simulink model "controller_sim"  (R2022a)
settings: Solver=ode1  StartTime=0.0  StopTime=10.0  FixedStep=0.010  RelTol=1e-5  AbsTol=1e-5
undefined symbols (not defined in the file or in its folder): c_d, c_dn, c_downbound, c_i, c_n, c_p, c_upbound, T0, T1, Td, Tg, Ti, Ts, Tsp, Tsp_delay, Tt
libraries: slpidlib x1
(part 1 of 3)
settings Model: Creator=baikp  LastModifiedBy=fxq001
settings SolverCC: AlgebraicLoopSolver=TrustRegion
settings DebuggingCC: UnconnectedInputMsg=warning  UnconnectedOutputMsg=warning  UnconnectedLineMsg=warning  SFMachineParentedDataDiag=warning
settings RTWCC: DLArmComputeVersion=19.05

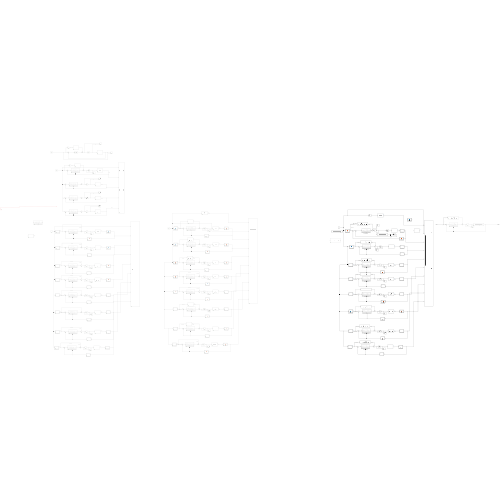
[thumbnail: Simulink's stored preview of the top-level diagram]
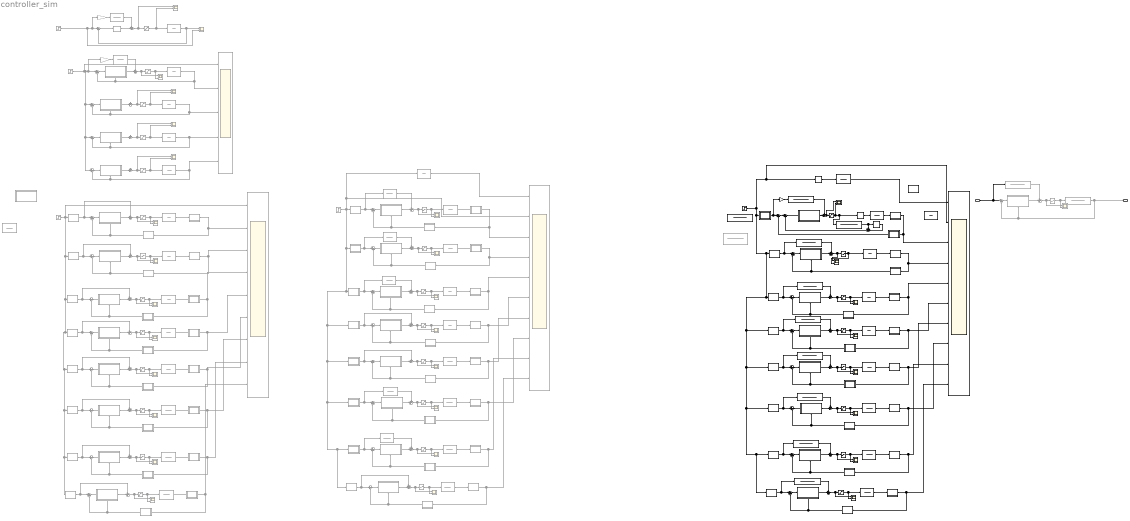
== system controller_sim ==
  In1 : Inport
  013throttle2wrpm1 : MATLAB Function  Commented=on  TreatAsAtomicUnit=on
  013throttle2wrpm2 : MATLAB Function  Commented=on  TreatAsAtomicUnit=on
  013throttle2wrpm3 : MATLAB Function  TreatAsAtomicUnit=on
  013wrpm2throttle2 : MATLAB Function  Commented=on  TreatAsAtomicUnit=on
  013wrpm2throttle3 : MATLAB Function  Commented=on  TreatAsAtomicUnit=on
  015throttle2wrpm1 : MATLAB Function  Commented=on  TreatAsAtomicUnit=on
  015throttle2wrpm2 : MATLAB Function  Commented=on  TreatAsAtomicUnit=on
  015throttle2wrpm3 : MATLAB Function  TreatAsAtomicUnit=on
  015wrpm2throttle1 : MATLAB Function  Commented=on  TreatAsAtomicUnit=on
  015wrpm2throttle4 : MATLAB Function  Commented=on  TreatAsAtomicUnit=on
  426throttle2wrpm1 : MATLAB Function  Commented=on  TreatAsAtomicUnit=on
  426throttle2wrpm2 : MATLAB Function  Commented=on  TreatAsAtomicUnit=on
  426throttle2wrpm3 : MATLAB Function  TreatAsAtomicUnit=on
  426wrpm2throttle2 : MATLAB Function  Commented=on  TreatAsAtomicUnit=on
  426wrpm2throttle3 : MATLAB Function  Commented=on  TreatAsAtomicUnit=on
  427throttle2wrpm1 : MATLAB Function  Commented=on  TreatAsAtomicUnit=on
  427throttle2wrpm2 : MATLAB Function  Commented=on  TreatAsAtomicUnit=on
  427throttle2wrpm3 : MATLAB Function  TreatAsAtomicUnit=on
  427wrpm2throttle1 : MATLAB Function  Commented=on  TreatAsAtomicUnit=on
  427wrpm2throttle10 : MATLAB Function  Commented=on  TreatAsAtomicUnit=on
  427wrpm2throttle11 : MATLAB Function  Commented=on  TreatAsAtomicUnit=on
  427wrpm2throttle12 : MATLAB Function  Commented=on  TreatAsAtomicUnit=on
  427wrpm2throttle13 : MATLAB Function  Commented=on  TreatAsAtomicUnit=on
  427wrpm2throttle14 : MATLAB Function  Commented=on  TreatAsAtomicUnit=on
  427wrpm2throttle15 : MATLAB Function  Commented=on  TreatAsAtomicUnit=on
  427wrpm2throttle16 : MATLAB Function  Commented=on  TreatAsAtomicUnit=on
  427wrpm2throttle17 : MATLAB Function  Commented=on  TreatAsAtomicUnit=on
  427wrpm2throttle18 : MATLAB Function  Commented=on  TreatAsAtomicUnit=on
  427wrpm2throttle19 : MATLAB Function  TreatAsAtomicUnit=on
  427wrpm2throttle2 : MATLAB Function  Commented=on  TreatAsAtomicUnit=on
  427wrpm2throttle20 : MATLAB Function  TreatAsAtomicUnit=on
  427wrpm2throttle21 : MATLAB Function  TreatAsAtomicUnit=on
  427wrpm2throttle22 : MATLAB Function  TreatAsAtomicUnit=on
  427wrpm2throttle23 : MATLAB Function  TreatAsAtomicUnit=on
  427wrpm2throttle24 : MATLAB Function  TreatAsAtomicUnit=on
  427wrpm2throttle25 : MATLAB Function  TreatAsAtomicUnit=on
  427wrpm2throttle26 : MATLAB Function  TreatAsAtomicUnit=on
  427wrpm2throttle27 : MATLAB Function  TreatAsAtomicUnit=on
  427wrpm2throttle28 : MATLAB Function  TreatAsAtomicUnit=on
  427wrpm2throttle29 : MATLAB Function  TreatAsAtomicUnit=on
  427wrpm2throttle3 : MATLAB Function  Commented=on  TreatAsAtomicUnit=on
  427wrpm2throttle30 : MATLAB Function  TreatAsAtomicUnit=on
  427wrpm2throttle31 : MATLAB Function  TreatAsAtomicUnit=on
  427wrpm2throttle32 : MATLAB Function  TreatAsAtomicUnit=on
  427wrpm2throttle33 : MATLAB Function  TreatAsAtomicUnit=on
  427wrpm2throttle34 : MATLAB Function  TreatAsAtomicUnit=on
  427wrpm2throttle4 : MATLAB Function  Commented=on  TreatAsAtomicUnit=on
  427wrpm2throttle5 : MATLAB Function  Commented=on  TreatAsAtomicUnit=on
  427wrpm2throttle6 : MATLAB Function  Commented=on  TreatAsAtomicUnit=on
  427wrpm2throttle7 : MATLAB Function  Commented=on  TreatAsAtomicUnit=on
  427wrpm2throttle8 : MATLAB Function  Commented=on  TreatAsAtomicUnit=on
  427wrpm2throttle9 : MATLAB Function  Commented=on  TreatAsAtomicUnit=on
  428throttle2wrpm1 : MATLAB Function  Commented=on  TreatAsAtomicUnit=on
  428throttle2wrpm2 : MATLAB Function  Commented=on  TreatAsAtomicUnit=on
  428throttle2wrpm3 : MATLAB Function  TreatAsAtomicUnit=on
  428throttle2wrpm4 : MATLAB Function  TreatAsAtomicUnit=on
  428wrpm2throttle2 : MATLAB Function  Commented=on  TreatAsAtomicUnit=on
  428wrpm2throttle3 : MATLAB Function  Commented=on  TreatAsAtomicUnit=on
  429throttle2wrpm1 : MATLAB Function  Commented=on  TreatAsAtomicUnit=on
  429throttle2wrpm2 : MATLAB Function  Commented=on  TreatAsAtomicUnit=on
  429throttle2wrpm3 : MATLAB Function  TreatAsAtomicUnit=on
  429wrpm2throttle1 : MATLAB Function  Commented=on  TreatAsAtomicUnit=on
  429wrpm2throttle4 : MATLAB Function  Commented=on  TreatAsAtomicUnit=on
  430throttle2wrpm1 : MATLAB Function  Commented=on  TreatAsAtomicUnit=on
  430throttle2wrpm2 : MATLAB Function  Commented=on  TreatAsAtomicUnit=on
  430throttle2wrpm3 : MATLAB Function  TreatAsAtomicUnit=on
  430wrpm2throttle2 : MATLAB Function  Commented=on  TreatAsAtomicUnit=on
  430wrpm2throttle3 : MATLAB Function  Commented=on  TreatAsAtomicUnit=on
  431throttle2wrpm : MATLAB Function  Commented=on  TreatAsAtomicUnit=on
  431throttle2wrpm1 : MATLAB Function  Commented=on  TreatAsAtomicUnit=on
  431throttle2wrpm2 : MATLAB Function  TreatAsAtomicUnit=on
  431wrpm2throttle : MATLAB Function  Commented=on  TreatAsAtomicUnit=on
  431wrpm2throttle1 : MATLAB Function  Commented=on  TreatAsAtomicUnit=on
  Discrete Transfer Fcn1 : DiscreteTransferFcn  Numerator=[Ts Ts]  Denominator=[(Ts+2*Tg) (Ts-2*Tg)]
  Discrete Transfer Fcn10 : DiscreteTransferFcn  Commented=on  Numerator=[Ts Ts]  Denominator=[(Ts+0.3) (Ts-0.3)]
  Discrete Transfer Fcn11 : DiscreteTransferFcn  Commented=on  Numerator=[Ts Ts]  Denominator=[(Ts+0.4) (Ts-0.4)]
  Discrete Transfer Fcn12 : DiscreteTransferFcn  Commented=on  Numerator=[(2*T0+Ts) (Ts-2*T0)]  Denominator=[(2*T1+Ts ) (Ts-2*T1)]
  Discrete Transfer Fcn{2..8,13} (8 alike) : DiscreteTransferFcn  Numerator=[Ts Ts]  Denominator=[(Ts+0.3) (Ts-0.3)]
  Discrete Transfer Fcn9 : DiscreteTransferFcn  Numerator=[Ts Ts]  Denominator=[(Ts+2*Tsp) (Ts-2*Tsp)]
  Gain : Gain  Commented=on  Gain=0.0012
  Gain1 : Gain  Commented=on  Gain=0.0012
  Gain2 : Gain  Gain=0.8
  PID Controller : slpidlib/PID Controller  Commented=on  Controller=PID  Form=Parallel  TimeDomain=Continuous-time  UseExternalTs=off  SampleTime=-1  IntegratorMethod=Forward Euler  FilterMethod=Forward Euler  ControllerParametersSource=internal  P=27.5*0.5  I=84.7*0.5  UseKiTs=off  D=2.2*0.5  N=100  UseFilter=on  TunerSelectOption=Transfer Function Based (PID Tuner App)  InitialConditionSource=internal  InitialConditionForIntegrator=0  InitialConditionForFilter=0  DifferentiatorICPrevScaledInput=0  ExternalReset=none  TrackingMode=off  Kt=1  LimitOutput=on  SatLimitsSource=internal  UpperSaturationLimit=200  LowerSaturationLimit=0  LinearizeAsGain=on  AntiWindupMode=back-calculation  Kb=4  POutMin=[]  POutMax=[]  IOutMin=[]  IOutMax=[]  DOutMin=[]  DOutMax=[]  NOutMin=[]  NOutMax=[]  SumOutMin=[]  SumOutMax=[]  SaturationOutMin=[]  SaturationOutMax=[]  PParamMin=[]  PParamMax=[]  IParamMin=[]  IParamMax=[]  DParamMin=[]  DParamMax=[]  NParamMin=[]  NParamMax=[]  KbParamMin=[]  KbParamMax=[]  KtParamMin=[]  KtParamMax=[]  KbOutMin=[]  KbOutMax=[]  KtOutMin=[]  KtOutMax=[]  IntegratorOutMin=[]  IntegratorOutMax=[]  FilterOutMin=[]  FilterOutMax=[]  SumI1OutMin=[]  SumI1OutMax=[]  SumI2OutMin=[]  SumI2OutMax=[]  SumI3OutMin=[]  SumI3OutMax=[]  SumI4OutMin=[]  SumI4OutMax=[]  SumDOutMin=[]  SumDOutMax=[]  DifferentiatorOutMin=[]  DifferentiatorOutMax=[]  FilterDiffOutCoefMin=[]  FilterDiffOutCoefMax=[]  ReciprocalOutMin=[]  ReciprocalOutMax=[]  SumDenOutMin=[]  SumDenOutMax=[]  SumNumOutMin=[]  SumNumOutMax=[]  DivideOutMin=[]  DivideOutMax=[]  UdiffTsProdOutMin=[]  UdiffTsProdOutMax=[]  NTsProdOutMin=[]  NTsProdOutMax=[]  UintegralTsProdOutMin=[]  UintegralTsProdOutMax=[]  UngainTsProdOutMin=[]  UngainTsProdOutMax=[]  IntegratorContinuousStateAttributes=''  IntegratorStateMustResolveToSignalObject=off  IntegratorRTWStateStorageClass=Auto  FilterContinuousStateAttributes=''  FilterStateMustResolveToSignalObject=off  FilterRTWStateStorageClass=Auto  ParallelPVariant=InternalParameters  IdealPVariant=Disabled  IVariant=InternalParameters  DVariant=InternalParameters  IntegratorVariant=Continuous  SatVariant=Enabled  AWVariant=BackCalculation  PCopyVariant=Disabled  TRVariant=Disabled  FdbkBlocksVariant=Forward  IdealPFdbkVariant=Disabled  SatFdbkVariant=Disabled  DerivativeFilterVariant=ContFilter  NVariant=InternalParameters  NCopyVariant=Disabled  FilterICVariant=InternalICsFilter  IntegratorICVariant=InternalICs  ExternalResetVariant=Disabled  TRSumVariant=Passthrough  SumFdbkVariant=Disabled  SumVariant=Sum_PID  TsampFilterVariant=InternalTs  TsampNgainVariant=Passthrough  TsampIntegralVariant=Passthrough  ExternalSaturationOutDataTypeStr=Inherit: Same as second input  aMode=0
  Saturation{,1..20,29} (22 alike) : Saturate  Commented=on  UpperLimit=1000  LowerLimit=0
  Saturation{21..28} (8 alike) : Saturate  UpperLimit=1000  LowerLimit=0
  Scope{,1,3..7,9..22,24,35} (23 alike) : Scope  Commented=on  NumInputPorts=2
  Scope2 : Scope  Commented=on  NumInputPorts=5
  Scope23 : Scope  Commented=on  NumInputPorts=10
  Scope{25..31,33} (8 alike) : Scope  NumInputPorts=2
  Scope32 : Scope  NumInputPorts=10
  Scope8 : Scope  Commented=on  NumInputPorts=9
  Step : Step  Commented=on  After=100  SampleTime=0
  Step1 : Step  Commented=on  After=100  SampleTime=0
  Step2 : Step  Commented=on  Before=7.5  After=8.5  SampleTime=0
  Step3 : Step  Commented=on  Time=5  Before=7.5  After=8.5  SampleTime=0
  Step4 : Step  Time=5  Before=7.5  After=8.5  SampleTime=0
  Subsystem : Subsystem  Commented=on
      settings: PortSchema="{\"entries\":[{\"content\":{\"sides\":[{\"content\":{\"connectorIds\":[\"In1\"]},\"type\":\"ConnectorPlacement.EquallySpacedRectSide\",\"uuid\":\"c21bf5a5-0def-4d0b-a33c-ffee9b3485af\"},{\"content\":{\"connectorIds\":[\"Out1\"],\"side\":\"RIGHT\"},\"type\":\"ConnectorPlacement.EquallySpacedRectSide\",\"uuid\":\"821ecc78-a01a-44e5-a9eb-88440e9f59ac\"},{\"content\":{\"connectorIds\":[],\"side\":\"TOP\"},\"type\":\"ConnectorPlacement.EquallySpacedRectSide\",\"uuid\":\"8999c1fd-a485-4668-b36c-e9eed9eb6d51\"},{\"content\":{\"connectorIds\":[\"In2\"],\"side\":\"BOTTOM\"},\"type\":\"ConnectorPlacement.EquallySpacedRectSide\",\"uuid\":\"a6e4704b-9925-4d06-9ffd-ba41902e8aa3\"},{\"content\":{\"connectorIds\":[],\"side\":\"HIDDEN\"},\"type\":\"ConnectorPlacement.EquallySpacedRectSide\",\"uuid\":\"86f54ccf-23de-43ab-be63-92a8881a04a3\"}]},\"type\":\"ConnectorPlacement.EquallySpacedConnector\",\"uuid\":\"5c8192db-99f5-4e0b-9632-6c54e7eb95e2\"}],\"packageUris\":[\"http://schema.mathworks.com/mf0/Connector/R2020b\"],\"version\":\"1.0\"}"
  Subsystem1 : Subsystem  Commented=on
      settings: PortSchema="{\"entries\":[{\"content\":{\"sides\":[{\"content\":{\"connectorIds\":[\"In1\"]},\"type\":\"ConnectorPlacement.EquallySpacedRectSide\",\"uuid\":\"c21bf5a5-0def-4d0b-a33c-ffee9b3485af\"},{\"content\":{\"connectorIds\":[\"Out1\"],\"side\":\"RIGHT\"},\"type\":\"ConnectorPlacement.EquallySpacedRectSide\",\"uuid\":\"821ecc78-a01a-44e5-a9eb-88440e9f59ac\"},{\"content\":{\"connectorIds\":[],\"side\":\"TOP\"},\"type\":\"ConnectorPlacement.EquallySpacedRectSide\",\"uuid\":\"8999c1fd-a485-4668-b36c-e9eed9eb6d51\"},{\"content\":{\"connectorIds\":[\"In2\"],\"side\":\"BOTTOM\"},\"type\":\"ConnectorPlacement.EquallySpacedRectSide\",\"uuid\":\"a6e4704b-9925-4d06-9ffd-ba41902e8aa3\"},{\"content\":{\"connectorIds\":[],\"side\":\"HIDDEN\"},\"type\":\"ConnectorPlacement.EquallySpacedRectSide\",\"uuid\":\"86f54ccf-23de-43ab-be63-92a8881a04a3\"}]},\"type\":\"ConnectorPlacement.EquallySpacedConnector\",\"uuid\":\"5c8192db-99f5-4e0b-9632-6c54e7eb95e2\"}],\"packageUris\":[\"http://schema.mathworks.com/mf0/Connector/R2020b\"],\"version\":\"1.0\"}"
  Subsystem10 : Subsystem  Commented=on
      settings: PortSchema="{\"entries\":[{\"content\":{\"sides\":[{\"content\":{\"connectorIds\":[\"In1\"]},\"type\":\"ConnectorPlacement.EquallySpacedRectSide\",\"uuid\":\"c21bf5a5-0def-4d0b-a33c-ffee9b3485af\"},{\"content\":{\"connectorIds\":[\"Out1\"],\"side\":\"RIGHT\"},\"type\":\"ConnectorPlacement.EquallySpacedRectSide\",\"uuid\":\"821ecc78-a01a-44e5-a9eb-88440e9f59ac\"},{\"content\":{\"connectorIds\":[],\"side\":\"TOP\"},\"type\":\"ConnectorPlacement.EquallySpacedRectSide\",\"uuid\":\"8999c1fd-a485-4668-b36c-e9eed9eb6d51\"},{\"content\":{\"connectorIds\":[\"In2\"],\"side\":\"BOTTOM\"},\"type\":\"ConnectorPlacement.EquallySpacedRectSide\",\"uuid\":\"a6e4704b-9925-4d06-9ffd-ba41902e8aa3\"},{\"content\":{\"connectorIds\":[],\"side\":\"HIDDEN\"},\"type\":\"ConnectorPlacement.EquallySpacedRectSide\",\"uuid\":\"86f54ccf-23de-43ab-be63-92a8881a04a3\"}]},\"type\":\"ConnectorPlacement.EquallySpacedConnector\",\"uuid\":\"5c8192db-99f5-4e0b-9632-6c54e7eb95e2\"}],\"packageUris\":[\"http://schema.mathworks.com/mf0/Connector/R2020b\"],\"version\":\"1.0\"}"
  Subsystem11 : Subsystem  Commented=on
      settings: PortSchema="{\"entries\":[{\"content\":{\"sides\":[{\"content\":{\"connectorIds\":[\"In1\"]},\"type\":\"ConnectorPlacement.EquallySpacedRectSide\",\"uuid\":\"c21bf5a5-0def-4d0b-a33c-ffee9b3485af\"},{\"content\":{\"connectorIds\":[\"Out1\"],\"side\":\"RIGHT\"},\"type\":\"ConnectorPlacement.EquallySpacedRectSide\",\"uuid\":\"821ecc78-a01a-44e5-a9eb-88440e9f59ac\"},{\"content\":{\"connectorIds\":[],\"side\":\"TOP\"},\"type\":\"ConnectorPlacement.EquallySpacedRectSide\",\"uuid\":\"8999c1fd-a485-4668-b36c-e9eed9eb6d51\"},{\"content\":{\"connectorIds\":[\"In2\"],\"side\":\"BOTTOM\"},\"type\":\"ConnectorPlacement.EquallySpacedRectSide\",\"uuid\":\"a6e4704b-9925-4d06-9ffd-ba41902e8aa3\"},{\"content\":{\"connectorIds\":[],\"side\":\"HIDDEN\"},\"type\":\"ConnectorPlacement.EquallySpacedRectSide\",\"uuid\":\"86f54ccf-23de-43ab-be63-92a8881a04a3\"}]},\"type\":\"ConnectorPlacement.EquallySpacedConnector\",\"uuid\":\"5c8192db-99f5-4e0b-9632-6c54e7eb95e2\"}],\"packageUris\":[\"http://schema.mathworks.com/mf0/Connector/R2020b\"],\"version\":\"1.0\"}"
  Subsystem12 : Subsystem  Commented=on
      settings: PortSchema="{\"entries\":[{\"content\":{\"sides\":[{\"content\":{\"connectorIds\":[\"In1\"]},\"type\":\"ConnectorPlacement.EquallySpacedRectSide\",\"uuid\":\"c21bf5a5-0def-4d0b-a33c-ffee9b3485af\"},{\"content\":{\"connectorIds\":[\"Out1\"],\"side\":\"RIGHT\"},\"type\":\"ConnectorPlacement.EquallySpacedRectSide\",\"uuid\":\"821ecc78-a01a-44e5-a9eb-88440e9f59ac\"},{\"content\":{\"connectorIds\":[],\"side\":\"TOP\"},\"type\":\"ConnectorPlacement.EquallySpacedRectSide\",\"uuid\":\"8999c1fd-a485-4668-b36c-e9eed9eb6d51\"},{\"content\":{\"connectorIds\":[\"In2\"],\"side\":\"BOTTOM\"},\"type\":\"ConnectorPlacement.EquallySpacedRectSide\",\"uuid\":\"a6e4704b-9925-4d06-9ffd-ba41902e8aa3\"},{\"content\":{\"connectorIds\":[],\"side\":\"HIDDEN\"},\"type\":\"ConnectorPlacement.EquallySpacedRectSide\",\"uuid\":\"86f54ccf-23de-43ab-be63-92a8881a04a3\"}]},\"type\":\"ConnectorPlacement.EquallySpacedConnector\",\"uuid\":\"5c8192db-99f5-4e0b-9632-6c54e7eb95e2\"}],\"packageUris\":[\"http://schema.mathworks.com/mf0/Connector/R2020b\"],\"version\":\"1.0\"}"
  Subsystem13 : Subsystem  Commented=on
      settings: PortSchema="{\"entries\":[{\"content\":{\"sides\":[{\"content\":{\"connectorIds\":[\"In1\"]},\"type\":\"ConnectorPlacement.EquallySpacedRectSide\",\"uuid\":\"c21bf5a5-0def-4d0b-a33c-ffee9b3485af\"},{\"content\":{\"connectorIds\":[\"Out1\"],\"side\":\"RIGHT\"},\"type\":\"ConnectorPlacement.EquallySpacedRectSide\",\"uuid\":\"821ecc78-a01a-44e5-a9eb-88440e9f59ac\"},{\"content\":{\"connectorIds\":[],\"side\":\"TOP\"},\"type\":\"ConnectorPlacement.EquallySpacedRectSide\",\"uuid\":\"8999c1fd-a485-4668-b36c-e9eed9eb6d51\"},{\"content\":{\"connectorIds\":[\"In2\"],\"side\":\"BOTTOM\"},\"type\":\"ConnectorPlacement.EquallySpacedRectSide\",\"uuid\":\"a6e4704b-9925-4d06-9ffd-ba41902e8aa3\"},{\"content\":{\"connectorIds\":[],\"side\":\"HIDDEN\"},\"type\":\"ConnectorPlacement.EquallySpacedRectSide\",\"uuid\":\"86f54ccf-23de-43ab-be63-92a8881a04a3\"}]},\"type\":\"ConnectorPlacement.EquallySpacedConnector\",\"uuid\":\"5c8192db-99f5-4e0b-9632-6c54e7eb95e2\"}],\"packageUris\":[\"http://schema.mathworks.com/mf0/Connector/R2020b\"],\"version\":\"1.0\"}"
  Subsystem14 : Subsystem  Commented=on
      settings: PortSchema="{\"entries\":[{\"content\":{\"sides\":[{\"content\":{\"connectorIds\":[\"In1\"]},\"type\":\"ConnectorPlacement.EquallySpacedRectSide\",\"uuid\":\"c21bf5a5-0def-4d0b-a33c-ffee9b3485af\"},{\"content\":{\"connectorIds\":[\"Out1\"],\"side\":\"RIGHT\"},\"type\":\"ConnectorPlacement.EquallySpacedRectSide\",\"uuid\":\"821ecc78-a01a-44e5-a9eb-88440e9f59ac\"},{\"content\":{\"connectorIds\":[],\"side\":\"TOP\"},\"type\":\"ConnectorPlacement.EquallySpacedRectSide\",\"uuid\":\"8999c1fd-a485-4668-b36c-e9eed9eb6d51\"},{\"content\":{\"connectorIds\":[\"In2\"],\"side\":\"BOTTOM\"},\"type\":\"ConnectorPlacement.EquallySpacedRectSide\",\"uuid\":\"a6e4704b-9925-4d06-9ffd-ba41902e8aa3\"},{\"content\":{\"connectorIds\":[],\"side\":\"HIDDEN\"},\"type\":\"ConnectorPlacement.EquallySpacedRectSide\",\"uuid\":\"86f54ccf-23de-43ab-be63-92a8881a04a3\"}]},\"type\":\"ConnectorPlacement.EquallySpacedConnector\",\"uuid\":\"5c8192db-99f5-4e0b-9632-6c54e7eb95e2\"}],\"packageUris\":[\"http://schema.mathworks.com/mf0/Connector/R2020b\"],\"version\":\"1.0\"}"
  Subsystem15 : Subsystem  Commented=on
      settings: PortSchema="{\"entries\":[{\"content\":{\"sides\":[{\"content\":{\"connectorIds\":[\"In1\"]},\"type\":\"ConnectorPlacement.EquallySpacedRectSide\",\"uuid\":\"c21bf5a5-0def-4d0b-a33c-ffee9b3485af\"},{\"content\":{\"connectorIds\":[\"Out1\"],\"side\":\"RIGHT\"},\"type\":\"ConnectorPlacement.EquallySpacedRectSide\",\"uuid\":\"821ecc78-a01a-44e5-a9eb-88440e9f59ac\"},{\"content\":{\"connectorIds\":[],\"side\":\"TOP\"},\"type\":\"ConnectorPlacement.EquallySpacedRectSide\",\"uuid\":\"8999c1fd-a485-4668-b36c-e9eed9eb6d51\"},{\"content\":{\"connectorIds\":[\"In2\"],\"side\":\"BOTTOM\"},\"type\":\"ConnectorPlacement.EquallySpacedRectSide\",\"uuid\":\"a6e4704b-9925-4d06-9ffd-ba41902e8aa3\"},{\"content\":{\"connectorIds\":[],\"side\":\"HIDDEN\"},\"type\":\"ConnectorPlacement.EquallySpacedRectSide\",\"uuid\":\"86f54ccf-23de-43ab-be63-92a8881a04a3\"}]},\"type\":\"ConnectorPlacement.EquallySpacedConnector\",\"uuid\":\"5c8192db-99f5-4e0b-9632-6c54e7eb95e2\"}],\"packageUris\":[\"http://schema.mathworks.com/mf0/Connector/R2020b\"],\"version\":\"1.0\"}"
  Subsystem16 : Subsystem  Commented=on
      settings: PortSchema="{\"entries\":[{\"content\":{\"sides\":[{\"content\":{\"connectorIds\":[\"In1\"]},\"type\":\"ConnectorPlacement.EquallySpacedRectSide\",\"uuid\":\"c21bf5a5-0def-4d0b-a33c-ffee9b3485af\"},{\"content\":{\"connectorIds\":[\"Out1\"],\"side\":\"RIGHT\"},\"type\":\"ConnectorPlacement.EquallySpacedRectSide\",\"uuid\":\"821ecc78-a01a-44e5-a9eb-88440e9f59ac\"},{\"content\":{\"connectorIds\":[],\"side\":\"TOP\"},\"type\":\"ConnectorPlacement.EquallySpacedRectSide\",\"uuid\":\"8999c1fd-a485-4668-b36c-e9eed9eb6d51\"},{\"content\":{\"connectorIds\":[\"In2\"],\"side\":\"BOTTOM\"},\"type\":\"ConnectorPlacement.EquallySpacedRectSide\",\"uuid\":\"a6e4704b-9925-4d06-9ffd-ba41902e8aa3\"},{\"content\":{\"connectorIds\":[],\"side\":\"HIDDEN\"},\"type\":\"ConnectorPlacement.EquallySpacedRectSide\",\"uuid\":\"86f54ccf-23de-43ab-be63-92a8881a04a3\"}]},\"type\":\"ConnectorPlacement.EquallySpacedConnector\",\"uuid\":\"5c8192db-99f5-4e0b-9632-6c54e7eb95e2\"}],\"packageUris\":[\"http://schema.mathworks.com/mf0/Connector/R2020b\"],\"version\":\"1.0\"}"
  Subsystem17 : Subsystem  Commented=on
      settings: PortSchema="{\"entries\":[{\"content\":{\"sides\":[{\"content\":{\"connectorIds\":[\"In1\"]},\"type\":\"ConnectorPlacement.EquallySpacedRectSide\",\"uuid\":\"c21bf5a5-0def-4d0b-a33c-ffee9b3485af\"},{\"content\":{\"connectorIds\":[\"Out1\"],\"side\":\"RIGHT\"},\"type\":\"ConnectorPlacement.EquallySpacedRectSide\",\"uuid\":\"821ecc78-a01a-44e5-a9eb-88440e9f59ac\"},{\"content\":{\"connectorIds\":[],\"side\":\"TOP\"},\"type\":\"ConnectorPlacement.EquallySpacedRectSide\",\"uuid\":\"8999c1fd-a485-4668-b36c-e9eed9eb6d51\"},{\"content\":{\"connectorIds\":[\"In2\"],\"side\":\"BOTTOM\"},\"type\":\"ConnectorPlacement.EquallySpacedRectSide\",\"uuid\":\"a6e4704b-9925-4d06-9ffd-ba41902e8aa3\"},{\"content\":{\"connectorIds\":[],\"side\":\"HIDDEN\"},\"type\":\"ConnectorPlacement.EquallySpacedRectSide\",\"uuid\":\"86f54ccf-23de-43ab-be63-92a8881a04a3\"}]},\"type\":\"ConnectorPlacement.EquallySpacedConnector\",\"uuid\":\"5c8192db-99f5-4e0b-9632-6c54e7eb95e2\"}],\"packageUris\":[\"http://schema.mathworks.com/mf0/Connector/R2020b\"],\"version\":\"1.0\"}"
  Subsystem18 : Subsystem  Commented=on
      settings: PortSchema="{\"entries\":[{\"content\":{\"sides\":[{\"content\":{\"connectorIds\":[\"In1\"]},\"type\":\"ConnectorPlacement.EquallySpacedRectSide\",\"uuid\":\"c21bf5a5-0def-4d0b-a33c-ffee9b3485af\"},{\"content\":{\"connectorIds\":[\"Out1\"],\"side\":\"RIGHT\"},\"type\":\"ConnectorPlacement.EquallySpacedRectSide\",\"uuid\":\"821ecc78-a01a-44e5-a9eb-88440e9f59ac\"},{\"content\":{\"connectorIds\":[],\"side\":\"TOP\"},\"type\":\"ConnectorPlacement.EquallySpacedRectSide\",\"uuid\":\"8999c1fd-a485-4668-b36c-e9eed9eb6d51\"},{\"content\":{\"connectorIds\":[\"In2\"],\"side\":\"BOTTOM\"},\"type\":\"ConnectorPlacement.EquallySpacedRectSide\",\"uuid\":\"a6e4704b-9925-4d06-9ffd-ba41902e8aa3\"},{\"content\":{\"connectorIds\":[],\"side\":\"HIDDEN\"},\"type\":\"ConnectorPlacement.EquallySpacedRectSide\",\"uuid\":\"86f54ccf-23de-43ab-be63-92a8881a04a3\"}]},\"type\":\"ConnectorPlacement.EquallySpacedConnector\",\"uuid\":\"5c8192db-99f5-4e0b-9632-6c54e7eb95e2\"}],\"packageUris\":[\"http://schema.mathworks.com/mf0/Connector/R2020b\"],\"version\":\"1.0\"}"
  Subsystem19 : Subsystem  Commented=on
      settings: PortSchema="{\"entries\":[{\"content\":{\"sides\":[{\"content\":{\"connectorIds\":[\"In1\"]},\"type\":\"ConnectorPlacement.EquallySpacedRectSide\",\"uuid\":\"c21bf5a5-0def-4d0b-a33c-ffee9b3485af\"},{\"content\":{\"connectorIds\":[\"Out1\"],\"side\":\"RIGHT\"},\"type\":\"ConnectorPlacement.EquallySpacedRectSide\",\"uuid\":\"821ecc78-a01a-44e5-a9eb-88440e9f59ac\"},{\"content\":{\"connectorIds\":[],\"side\":\"TOP\"},\"type\":\"ConnectorPlacement.EquallySpacedRectSide\",\"uuid\":\"8999c1fd-a485-4668-b36c-e9eed9eb6d51\"},{\"content\":{\"connectorIds\":[\"In2\"],\"side\":\"BOTTOM\"},\"type\":\"ConnectorPlacement.EquallySpacedRectSide\",\"uuid\":\"a6e4704b-9925-4d06-9ffd-ba41902e8aa3\"},{\"content\":{\"connectorIds\":[],\"side\":\"HIDDEN\"},\"type\":\"ConnectorPlacement.EquallySpacedRectSide\",\"uuid\":\"86f54ccf-23de-43ab-be63-92a8881a04a3\"}]},\"type\":\"ConnectorPlacement.EquallySpacedConnector\",\"uuid\":\"5c8192db-99f5-4e0b-9632-6c54e7eb95e2\"}],\"packageUris\":[\"http://schema.mathworks.com/mf0/Connector/R2020b\"],\"version\":\"1.0\"}"
  Subsystem2 : Subsystem  Commented=on
      settings: PortSchema="{\"entries\":[{\"content\":{\"sides\":[{\"content\":{\"connectorIds\":[\"In1\"]},\"type\":\"ConnectorPlacement.EquallySpacedRectSide\",\"uuid\":\"c21bf5a5-0def-4d0b-a33c-ffee9b3485af\"},{\"content\":{\"connectorIds\":[\"Out1\"],\"side\":\"RIGHT\"},\"type\":\"ConnectorPlacement.EquallySpacedRectSide\",\"uuid\":\"821ecc78-a01a-44e5-a9eb-88440e9f59ac\"},{\"content\":{\"connectorIds\":[],\"side\":\"TOP\"},\"type\":\"ConnectorPlacement.EquallySpacedRectSide\",\"uuid\":\"8999c1fd-a485-4668-b36c-e9eed9eb6d51\"},{\"content\":{\"connectorIds\":[\"In2\"],\"side\":\"BOTTOM\"},\"type\":\"ConnectorPlacement.EquallySpacedRectSide\",\"uuid\":\"a6e4704b-9925-4d06-9ffd-ba41902e8aa3\"},{\"content\":{\"connectorIds\":[],\"side\":\"HIDDEN\"},\"type\":\"ConnectorPlacement.EquallySpacedRectSide\",\"uuid\":\"86f54ccf-23de-43ab-be63-92a8881a04a3\"}]},\"type\":\"ConnectorPlacement.EquallySpacedConnector\",\"uuid\":\"5c8192db-99f5-4e0b-9632-6c54e7eb95e2\"}],\"packageUris\":[\"http://schema.mathworks.com/mf0/Connector/R2020b\"],\"version\":\"1.0\"}"
  Subsystem22 : Subsystem  Commented=on
      settings: PortSchema="{\"entries\":[{\"content\":{\"sides\":[{\"content\":{\"connectorIds\":[\"In1\"]},\"type\":\"ConnectorPlacement.EquallySpacedRectSide\",\"uuid\":\"c21bf5a5-0def-4d0b-a33c-ffee9b3485af\"},{\"content\":{\"connectorIds\":[\"Out1\"],\"side\":\"RIGHT\"},\"type\":\"ConnectorPlacement.EquallySpacedRectSide\",\"uuid\":\"821ecc78-a01a-44e5-a9eb-88440e9f59ac\"},{\"content\":{\"connectorIds\":[],\"side\":\"TOP\"},\"type\":\"ConnectorPlacement.EquallySpacedRectSide\",\"uuid\":\"8999c1fd-a485-4668-b36c-e9eed9eb6d51\"},{\"content\":{\"connectorIds\":[\"In2\"],\"side\":\"BOTTOM\"},\"type\":\"ConnectorPlacement.EquallySpacedRectSide\",\"uuid\":\"a6e4704b-9925-4d06-9ffd-ba41902e8aa3\"},{\"content\":{\"connectorIds\":[],\"side\":\"HIDDEN\"},\"type\":\"ConnectorPlacement.EquallySpacedRectSide\",\"uuid\":\"86f54ccf-23de-43ab-be63-92a8881a04a3\"}]},\"type\":\"ConnectorPlacement.EquallySpacedConnector\",\"uuid\":\"5c8192db-99f5-4e0b-9632-6c54e7eb95e2\"}],\"packageUris\":[\"http://schema.mathworks.com/mf0/Connector/R2020b\"],\"version\":\"1.0\"}"
  Subsystem3 : Subsystem  Commented=on
      settings: PortSchema="{\"entries\":[{\"content\":{\"sides\":[{\"content\":{\"connectorIds\":[\"In1\"]},\"type\":\"ConnectorPlacement.EquallySpacedRectSide\",\"uuid\":\"c21bf5a5-0def-4d0b-a33c-ffee9b3485af\"},{\"content\":{\"connectorIds\":[\"Out1\"],\"side\":\"RIGHT\"},\"type\":\"ConnectorPlacement.EquallySpacedRectSide\",\"uuid\":\"821ecc78-a01a-44e5-a9eb-88440e9f59ac\"},{\"content\":{\"connectorIds\":[],\"side\":\"TOP\"},\"type\":\"ConnectorPlacement.EquallySpacedRectSide\",\"uuid\":\"8999c1fd-a485-4668-b36c-e9eed9eb6d51\"},{\"content\":{\"connectorIds\":[\"In2\"],\"side\":\"BOTTOM\"},\"type\":\"ConnectorPlacement.EquallySpacedRectSide\",\"uuid\":\"a6e4704b-9925-4d06-9ffd-ba41902e8aa3\"},{\"content\":{\"connectorIds\":[],\"side\":\"HIDDEN\"},\"type\":\"ConnectorPlacement.EquallySpacedRectSide\",\"uuid\":\"86f54ccf-23de-43ab-be63-92a8881a04a3\"}]},\"type\":\"ConnectorPlacement.EquallySpacedConnector\",\"uuid\":\"5c8192db-99f5-4e0b-9632-6c54e7eb95e2\"}],\"packageUris\":[\"http://schema.mathworks.com/mf0/Connector/R2020b\"],\"version\":\"1.0\"}"
  Subsystem4 : Subsystem  Commented=on
      settings: PortSchema="{\"entries\":[{\"content\":{\"sides\":[{\"content\":{\"connectorIds\":[\"In1\"]},\"type\":\"ConnectorPlacement.EquallySpacedRectSide\",\"uuid\":\"c21bf5a5-0def-4d0b-a33c-ffee9b3485af\"},{\"content\":{\"connectorIds\":[\"Out1\"],\"side\":\"RIGHT\"},\"type\":\"ConnectorPlacement.EquallySpacedRectSide\",\"uuid\":\"821ecc78-a01a-44e5-a9eb-88440e9f59ac\"},{\"content\":{\"connectorIds\":[],\"side\":\"TOP\"},\"type\":\"ConnectorPlacement.EquallySpacedRectSide\",\"uuid\":\"8999c1fd-a485-4668-b36c-e9eed9eb6d51\"},{\"content\":{\"connectorIds\":[\"In2\"],\"side\":\"BOTTOM\"},\"type\":\"ConnectorPlacement.EquallySpacedRectSide\",\"uuid\":\"a6e4704b-9925-4d06-9ffd-ba41902e8aa3\"},{\"content\":{\"connectorIds\":[],\"side\":\"HIDDEN\"},\"type\":\"ConnectorPlacement.EquallySpacedRectSide\",\"uuid\":\"86f54ccf-23de-43ab-be63-92a8881a04a3\"}]},\"type\":\"ConnectorPlacement.EquallySpacedConnector\",\"uuid\":\"5c8192db-99f5-4e0b-9632-6c54e7eb95e2\"}],\"packageUris\":[\"http://schema.mathworks.com/mf0/Connector/R2020b\"],\"version\":\"1.0\"}"
  Subsystem5 : Subsystem  Commented=on
      settings: PortSchema="{\"entries\":[{\"content\":{\"sides\":[{\"content\":{\"connectorIds\":[\"In1\"]},\"type\":\"ConnectorPlacement.EquallySpacedRectSide\",\"uuid\":\"c21bf5a5-0def-4d0b-a33c-ffee9b3485af\"},{\"content\":{\"connectorIds\":[\"Out1\"],\"side\":\"RIGHT\"},\"type\":\"ConnectorPlacement.EquallySpacedRectSide\",\"uuid\":\"821ecc78-a01a-44e5-a9eb-88440e9f59ac\"},{\"content\":{\"connectorIds\":[],\"side\":\"TOP\"},\"type\":\"ConnectorPlacement.EquallySpacedRectSide\",\"uuid\":\"8999c1fd-a485-4668-b36c-e9eed9eb6d51\"},{\"content\":{\"connectorIds\":[\"In2\"],\"side\":\"BOTTOM\"},\"type\":\"ConnectorPlacement.EquallySpacedRectSide\",\"uuid\":\"a6e4704b-9925-4d06-9ffd-ba41902e8aa3\"},{\"content\":{\"connectorIds\":[],\"side\":\"HIDDEN\"},\"type\":\"ConnectorPlacement.EquallySpacedRectSide\",\"uuid\":\"86f54ccf-23de-43ab-be63-92a8881a04a3\"}]},\"type\":\"ConnectorPlacement.EquallySpacedConnector\",\"uuid\":\"5c8192db-99f5-4e0b-9632-6c54e7eb95e2\"}],\"packageUris\":[\"http://schema.mathworks.com/mf0/Connector/R2020b\"],\"version\":\"1.0\"}"
  Subsystem6 : Subsystem  Commented=on
      settings: PortSchema="{\"entries\":[{\"content\":{\"sides\":[{\"content\":{\"connectorIds\":[\"In1\"]},\"type\":\"ConnectorPlacement.EquallySpacedRectSide\",\"uuid\":\"c21bf5a5-0def-4d0b-a33c-ffee9b3485af\"},{\"content\":{\"connectorIds\":[\"Out1\"],\"side\":\"RIGHT\"},\"type\":\"ConnectorPlacement.EquallySpacedRectSide\",\"uuid\":\"821ecc78-a01a-44e5-a9eb-88440e9f59ac\"},{\"content\":{\"connectorIds\":[],\"side\":\"TOP\"},\"type\":\"ConnectorPlacement.EquallySpacedRectSide\",\"uuid\":\"8999c1fd-a485-4668-b36c-e9eed9eb6d51\"},{\"content\":{\"connectorIds\":[\"In2\"],\"side\":\"BOTTOM\"},\"type\":\"ConnectorPlacement.EquallySpacedRectSide\",\"uuid\":\"a6e4704b-9925-4d06-9ffd-ba41902e8aa3\"},{\"content\":{\"connectorIds\":[],\"side\":\"HIDDEN\"},\"type\":\"ConnectorPlacement.EquallySpacedRectSide\",\"uuid\":\"86f54ccf-23de-43ab-be63-92a8881a04a3\"}]},\"type\":\"ConnectorPlacement.EquallySpacedConnector\",\"uuid\":\"5c8192db-99f5-4e0b-9632-6c54e7eb95e2\"}],\"packageUris\":[\"http://schema.mathworks.com/mf0/Connector/R2020b\"],\"version\":\"1.0\"}"
  Subsystem7 : Subsystem  Commented=on
      settings: PortSchema="{\"entries\":[{\"content\":{\"sides\":[{\"content\":{\"connectorIds\":[\"In1\"]},\"type\":\"ConnectorPlacement.EquallySpacedRectSide\",\"uuid\":\"c21bf5a5-0def-4d0b-a33c-ffee9b3485af\"},{\"content\":{\"connectorIds\":[\"Out1\"],\"side\":\"RIGHT\"},\"type\":\"ConnectorPlacement.EquallySpacedRectSide\",\"uuid\":\"821ecc78-a01a-44e5-a9eb-88440e9f59ac\"},{\"content\":{\"connectorIds\":[],\"side\":\"TOP\"},\"type\":\"ConnectorPlacement.EquallySpacedRectSide\",\"uuid\":\"8999c1fd-a485-4668-b36c-e9eed9eb6d51\"},{\"content\":{\"connectorIds\":[\"In2\"],\"side\":\"BOTTOM\"},\"type\":\"ConnectorPlacement.EquallySpacedRectSide\",\"uuid\":\"a6e4704b-9925-4d06-9ffd-ba41902e8aa3\"},{\"content\":{\"connectorIds\":[],\"side\":\"HIDDEN\"},\"type\":\"ConnectorPlacement.EquallySpacedRectSide\",\"uuid\":\"86f54ccf-23de-43ab-be63-92a8881a04a3\"}]},\"type\":\"ConnectorPlacement.EquallySpacedConnector\",\"uuid\":\"5c8192db-99f5-4e0b-9632-6c54e7eb95e2\"}],\"packageUris\":[\"http://schema.mathworks.com/mf0/Connector/R2020b\"],\"version\":\"1.0\"}"
  Subsystem8 : Subsystem  Commented=on
      settings: PortSchema="{\"entries\":[{\"content\":{\"sides\":[{\"content\":{\"connectorIds\":[\"In1\"]},\"type\":\"ConnectorPlacement.EquallySpacedRectSide\",\"uuid\":\"c21bf5a5-0def-4d0b-a33c-ffee9b3485af\"},{\"content\":{\"connectorIds\":[\"Out1\"],\"side\":\"RIGHT\"},\"type\":\"ConnectorPlacement.EquallySpacedRectSide\",\"uuid\":\"821ecc78-a01a-44e5-a9eb-88440e9f59ac\"},{\"content\":{\"connectorIds\":[],\"side\":\"TOP\"},\"type\":\"ConnectorPlacement.EquallySpacedRectSide\",\"uuid\":\"8999c1fd-a485-4668-b36c-e9eed9eb6d51\"},{\"content\":{\"connectorIds\":[\"In2\"],\"side\":\"BOTTOM\"},\"type\":\"ConnectorPlacement.EquallySpacedRectSide\",\"uuid\":\"a6e4704b-9925-4d06-9ffd-ba41902e8aa3\"},{\"content\":{\"connectorIds\":[],\"side\":\"HIDDEN\"},\"type\":\"ConnectorPlacement.EquallySpacedRectSide\",\"uuid\":\"86f54ccf-23de-43ab-be63-92a8881a04a3\"}]},\"type\":\"ConnectorPlacement.EquallySpacedConnector\",\"uuid\":\"5c8192db-99f5-4e0b-9632-6c54e7eb95e2\"}],\"packageUris\":[\"http://schema.mathworks.com/mf0/Connector/R2020b\"],\"version\":\"1.0\"}"
  Subsystem9 : Subsystem  Commented=on
      settings: PortSchema="{\"entries\":[{\"content\":{\"sides\":[{\"content\":{\"connectorIds\":[\"In1\"]},\"type\":\"ConnectorPlacement.EquallySpacedRectSide\",\"uuid\":\"c21bf5a5-0def-4d0b-a33c-ffee9b3485af\"},{\"content\":{\"connectorIds\":[\"Out1\"],\"side\":\"RIGHT\"},\"type\":\"ConnectorPlacement.EquallySpacedRectSide\",\"uuid\":\"821ecc78-a01a-44e5-a9eb-88440e9f59ac\"},{\"content\":{\"connectorIds\":[],\"side\":\"TOP\"},\"type\":\"ConnectorPlacement.EquallySpacedRectSide\",\"uuid\":\"8999c1fd-a485-4668-b36c-e9eed9eb6d51\"},{\"content\":{\"connectorIds\":[\"In2\"],\"side\":\"BOTTOM\"},\"type\":\"ConnectorPlacement.EquallySpacedRectSide\",\"uuid\":\"a6e4704b-9925-4d06-9ffd-ba41902e8aa3\"},{\"content\":{\"connectorIds\":[],\"side\":\"HIDDEN\"},\"type\":\"ConnectorPlacement.EquallySpacedRectSide\",\"uuid\":\"86f54ccf-23de-43ab-be63-92a8881a04a3\"}]},\"type\":\"ConnectorPlacement.EquallySpacedConnector\",\"uuid\":\"5c8192db-99f5-4e0b-9632-6c54e7eb95e2\"}],\"packageUris\":[\"http://schema.mathworks.com/mf0/Connector/R2020b\"],\"version\":\"1.0\"}"
  Sum{,3,5,7,9,11,13,15,17,19,21,23,25,27,29,31,33,35,37,39,41,59} (22 alike) : Sum  Commented=on  Inputs=|+-
  Sum{1..2,4,6,8,10,12,14,16,18,20,22,24,26,28,30,32,34,36,38,40,58} (22 alike) : Sum  Commented=on  Inputs=++|
  Sum{42,44,46,48,50,52,54,56} (8 alike) : Sum  Inputs=++|
  Sum{43,45,47,49,51,53,55,57,61} (9 alike) : Sum  Inputs=|+-
  Sum60 : Sum  Inputs=+-|
  Transfer Fcn{,1,7,22} (4 alike) : TransferFcn  Commented=on  Numerator=[5]  Denominator=[1 5]
  Transfer Fcn10 : TransferFcn  Commented=on  Numerator=[4]  Denominator=[1 4]
  Transfer Fcn{6,11..12,18} (4 alike) : TransferFcn  Commented=on  Numerator=[2.5]  Denominator=[1 2.5]
  Transfer Fcn{13..15,19..21} (6 alike) : TransferFcn  Commented=on  Denominator=[1/2.3 1]
  Transfer Fcn16 : TransferFcn  Commented=on  Numerator=[4]  Denominator=[1 4]
  Transfer Fcn17 : TransferFcn  Commented=on  Numerator=[2]  Denominator=[1 2]
  Transfer Fcn2 : TransferFcn  Commented=on  Numerator=[0.2 1]  Denominator=[0.05 1]
  Transfer Fcn23 : TransferFcn  Commented=on  Numerator=[2]  Denominator=[1 2]
  Transfer Fcn24 : TransferFcn  Commented=on  Numerator=[2]  Denominator=[1 2]
  Transfer Fcn{25..29} (5 alike) : TransferFcn  Commented=on  Denominator=[0.15 1]
  Transfer Fcn3 : TransferFcn  Commented=on  Numerator=[0.2 1]  Denominator=[0.05 1]
  Transfer Fcn30 : TransferFcn  Numerator=[4]  Denominator=[1 4]
  Transfer Fcn31 : TransferFcn  Numerator=[2]  Denominator=[1 2]
  Transfer Fcn32 : TransferFcn  Numerator=[2.5]  Denominator=[1 2.5]
  Transfer Fcn33 : TransferFcn  Denominator=[1/2.3 1]
  Transfer Fcn34 : TransferFcn  Denominator=[1/2.3 1]
  Transfer Fcn35 : TransferFcn  Denominator=[1/2.3 1]
  Transfer Fcn36 : TransferFcn  Denominator=[0.4 1]
  Transfer Fcn37 : TransferFcn  Numerator=[2]  Denominator=[1 2]
  Transfer Fcn38 : TransferFcn  Denominator=[0.22 1]
  Transfer Fcn39 : TransferFcn  Numerator=[5]  Denominator=[1 5]
  Transfer Fcn4 : TransferFcn  Commented=on  Numerator=[7]  Denominator=[1 7]
  Transfer Fcn5 : TransferFcn  Commented=on  Numerator=[3]  Denominator=[1 3]
  Transfer Fcn8 : TransferFcn  Commented=on  Numerator=[2 1]  Denominator=[0.01 1]
  Transfer Fcn9 : TransferFcn  Commented=on  Numerator=[3]  Denominator=[1 3]
  Transport Delay1 : TransportDelay  DelayTime=Tsp_delay
  Transport Delay2 : TransportDelay  DelayTime=0.15
  Transport Delay3 : TransportDelay  DelayTime=0.15
  discreteController1 : Subsystem
      settings: PortSchema="{\"entries\":[{\"content\":{\"sides\":[{\"content\":{\"connectorIds\":[\"In1\"]},\"type\":\"ConnectorPlacement.EquallySpacedRectSide\",\"uuid\":\"c21bf5a5-0def-4d0b-a33c-ffee9b3485af\"},{\"content\":{\"connectorIds\":[\"Out1\"],\"side\":\"RIGHT\"},\"type\":\"ConnectorPlacement.EquallySpacedRectSide\",\"uuid\":\"821ecc78-a01a-44e5-a9eb-88440e9f59ac\"},{\"content\":{\"connectorIds\":[],\"side\":\"TOP\"},\"type\":\"ConnectorPlacement.EquallySpacedRectSide\",\"uuid\":\"8999c1fd-a485-4668-b36c-e9eed9eb6d51\"},{\"content\":{\"connectorIds\":[\"In2\"],\"side\":\"BOTTOM\"},\"type\":\"ConnectorPlacement.EquallySpacedRectSide\",\"uuid\":\"a6e4704b-9925-4d06-9ffd-ba41902e8aa3\"},{\"content\":{\"connectorIds\":[],\"side\":\"HIDDEN\"},\"type\":\"ConnectorPlacement.EquallySpacedRectSide\",\"uuid\":\"86f54ccf-23de-43ab-be63-92a8881a04a3\"}]},\"type\":\"ConnectorPlacement.EquallySpacedConnector\",\"uuid\":\"5c8192db-99f5-4e0b-9632-6c54e7eb95e2\"}],\"packageUris\":[\"http://schema.mathworks.com/mf0/Connector/R2020b\"],\"version\":\"1.0\"}"
  discreteController10 : Subsystem  Commented=on
      settings: PortSchema="{\"entries\":[{\"content\":{\"sides\":[{\"content\":{\"connectorIds\":[\"In1\"]},\"type\":\"ConnectorPlacement.EquallySpacedRectSide\",\"uuid\":\"c21bf5a5-0def-4d0b-a33c-ffee9b3485af\"},{\"content\":{\"connectorIds\":[\"Out1\"],\"side\":\"RIGHT\"},\"type\":\"ConnectorPlacement.EquallySpacedRectSide\",\"uuid\":\"821ecc78-a01a-44e5-a9eb-88440e9f59ac\"},{\"content\":{\"connectorIds\":[],\"side\":\"TOP\"},\"type\":\"ConnectorPlacement.EquallySpacedRectSide\",\"uuid\":\"8999c1fd-a485-4668-b36c-e9eed9eb6d51\"},{\"content\":{\"connectorIds\":[\"In2\"],\"side\":\"BOTTOM\"},\"type\":\"ConnectorPlacement.EquallySpacedRectSide\",\"uuid\":\"a6e4704b-9925-4d06-9ffd-ba41902e8aa3\"},{\"content\":{\"connectorIds\":[],\"side\":\"HIDDEN\"},\"type\":\"ConnectorPlacement.EquallySpacedRectSide\",\"uuid\":\"86f54ccf-23de-43ab-be63-92a8881a04a3\"}]},\"type\":\"ConnectorPlacement.EquallySpacedConnector\",\"uuid\":\"5c8192db-99f5-4e0b-9632-6c54e7eb95e2\"}],\"packageUris\":[\"http://schema.mathworks.com/mf0/Connector/R2020b\"],\"version\":\"1.0\"}"
  discreteController2 : Subsystem
      settings: PortSchema="{\"entries\":[{\"content\":{\"sides\":[{\"content\":{\"connectorIds\":[\"In1\"]},\"type\":\"ConnectorPlacement.EquallySpacedRectSide\",\"uuid\":\"c21bf5a5-0def-4d0b-a33c-ffee9b3485af\"},{\"content\":{\"connectorIds\":[\"Out1\"],\"side\":\"RIGHT\"},\"type\":\"ConnectorPlacement.EquallySpacedRectSide\",\"uuid\":\"821ecc78-a01a-44e5-a9eb-88440e9f59ac\"},{\"content\":{\"connectorIds\":[],\"side\":\"TOP\"},\"type\":\"ConnectorPlacement.EquallySpacedRectSide\",\"uuid\":\"8999c1fd-a485-4668-b36c-e9eed9eb6d51\"},{\"content\":{\"connectorIds\":[\"In2\"],\"side\":\"BOTTOM\"},\"type\":\"ConnectorPlacement.EquallySpacedRectSide\",\"uuid\":\"a6e4704b-9925-4d06-9ffd-ba41902e8aa3\"},{\"content\":{\"connectorIds\":[],\"side\":\"HIDDEN\"},\"type\":\"ConnectorPlacement.EquallySpacedRectSide\",\"uuid\":\"86f54ccf-23de-43ab-be63-92a8881a04a3\"}]},\"type\":\"ConnectorPlacement.EquallySpacedConnector\",\"uuid\":\"5c8192db-99f5-4e0b-9632-6c54e7eb95e2\"}],\"packageUris\":[\"http://schema.mathworks.com/mf0/Connector/R2020b\"],\"version\":\"1.0\"}"
  discreteController3 : Subsystem
      settings: PortSchema="{\"entries\":[{\"content\":{\"sides\":[{\"content\":{\"connectorIds\":[\"In1\"]},\"type\":\"ConnectorPlacement.EquallySpacedRectSide\",\"uuid\":\"c21bf5a5-0def-4d0b-a33c-ffee9b3485af\"},{\"content\":{\"connectorIds\":[\"Out1\"],\"side\":\"RIGHT\"},\"type\":\"ConnectorPlacement.EquallySpacedRectSide\",\"uuid\":\"821ecc78-a01a-44e5-a9eb-88440e9f59ac\"},{\"content\":{\"connectorIds\":[],\"side\":\"TOP\"},\"type\":\"ConnectorPlacement.EquallySpacedRectSide\",\"uuid\":\"8999c1fd-a485-4668-b36c-e9eed9eb6d51\"},{\"content\":{\"connectorIds\":[\"In2\"],\"side\":\"BOTTOM\"},\"type\":\"ConnectorPlacement.EquallySpacedRectSide\",\"uuid\":\"a6e4704b-9925-4d06-9ffd-ba41902e8aa3\"},{\"content\":{\"connectorIds\":[],\"side\":\"HIDDEN\"},\"type\":\"ConnectorPlacement.EquallySpacedRectSide\",\"uuid\":\"86f54ccf-23de-43ab-be63-92a8881a04a3\"}]},\"type\":\"ConnectorPlacement.EquallySpacedConnector\",\"uuid\":\"5c8192db-99f5-4e0b-9632-6c54e7eb95e2\"}],\"packageUris\":[\"http://schema.mathworks.com/mf0/Connector/R2020b\"],\"version\":\"1.0\"}"
  discreteController4 : Subsystem
      settings: PortSchema="{\"entries\":[{\"content\":{\"sides\":[{\"content\":{\"connectorIds\":[\"In1\"]},\"type\":\"ConnectorPlacement.EquallySpacedRectSide\",\"uuid\":\"c21bf5a5-0def-4d0b-a33c-ffee9b3485af\"},{\"content\":{\"connectorIds\":[\"Out1\"],\"side\":\"RIGHT\"},\"type\":\"ConnectorPlacement.EquallySpacedRectSide\",\"uuid\":\"821ecc78-a01a-44e5-a9eb-88440e9f59ac\"},{\"content\":{\"connectorIds\":[],\"side\":\"TOP\"},\"type\":\"ConnectorPlacement.EquallySpacedRectSide\",\"uuid\":\"8999c1fd-a485-4668-b36c-e9eed9eb6d51\"},{\"content\":{\"connectorIds\":[\"In2\"],\"side\":\"BOTTOM\"},\"type\":\"ConnectorPlacement.EquallySpacedRectSide\",\"uuid\":\"a6e4704b-9925-4d06-9ffd-ba41902e8aa3\"},{\"content\":{\"connectorIds\":[],\"side\":\"HIDDEN\"},\"type\":\"ConnectorPlacement.EquallySpacedRectSide\",\"uuid\":\"86f54ccf-23de-43ab-be63-92a8881a04a3\"}]},\"type\":\"ConnectorPlacement.EquallySpacedConnector\",\"uuid\":\"5c8192db-99f5-4e0b-9632-6c54e7eb95e2\"}],\"packageUris\":[\"http://schema.mathworks.com/mf0/Connector/R2020b\"],\"version\":\"1.0\"}"
  discreteController5 : Subsystem
      settings: PortSchema="{\"entries\":[{\"content\":{\"sides\":[{\"content\":{\"connectorIds\":[\"In1\"]},\"type\":\"ConnectorPlacement.EquallySpacedRectSide\",\"uuid\":\"c21bf5a5-0def-4d0b-a33c-ffee9b3485af\"},{\"content\":{\"connectorIds\":[\"Out1\"],\"side\":\"RIGHT\"},\"type\":\"ConnectorPlacement.EquallySpacedRectSide\",\"uuid\":\"821ecc78-a01a-44e5-a9eb-88440e9f59ac\"},{\"content\":{\"connectorIds\":[],\"side\":\"TOP\"},\"type\":\"ConnectorPlacement.EquallySpacedRectSide\",\"uuid\":\"8999c1fd-a485-4668-b36c-e9eed9eb6d51\"},{\"content\":{\"connectorIds\":[\"In2\"],\"side\":\"BOTTOM\"},\"type\":\"ConnectorPlacement.EquallySpacedRectSide\",\"uuid\":\"a6e4704b-9925-4d06-9ffd-ba41902e8aa3\"},{\"content\":{\"connectorIds\":[],\"side\":\"HIDDEN\"},\"type\":\"ConnectorPlacement.EquallySpacedRectSide\",\"uuid\":\"86f54ccf-23de-43ab-be63-92a8881a04a3\"}]},\"type\":\"ConnectorPlacement.EquallySpacedConnector\",\"uuid\":\"5c8192db-99f5-4e0b-9632-6c54e7eb95e2\"}],\"packageUris\":[\"http://schema.mathworks.com/mf0/Connector/R2020b\"],\"version\":\"1.0\"}"
  discreteController6 : Subsystem
      settings: PortSchema="{\"entries\":[{\"content\":{\"sides\":[{\"content\":{\"connectorIds\":[\"In1\"]},\"type\":\"ConnectorPlacement.EquallySpacedRectSide\",\"uuid\":\"c21bf5a5-0def-4d0b-a33c-ffee9b3485af\"},{\"content\":{\"connectorIds\":[\"Out1\"],\"side\":\"RIGHT\"},\"type\":\"ConnectorPlacement.EquallySpacedRectSide\",\"uuid\":\"821ecc78-a01a-44e5-a9eb-88440e9f59ac\"},{\"content\":{\"connectorIds\":[],\"side\":\"TOP\"},\"type\":\"ConnectorPlacement.EquallySpacedRectSide\",\"uuid\":\"8999c1fd-a485-4668-b36c-e9eed9eb6d51\"},{\"content\":{\"connectorIds\":[\"In2\"],\"side\":\"BOTTOM\"},\"type\":\"ConnectorPlacement.EquallySpacedRectSide\",\"uuid\":\"a6e4704b-9925-4d06-9ffd-ba41902e8aa3\"},{\"content\":{\"connectorIds\":[],\"side\":\"HIDDEN\"},\"type\":\"ConnectorPlacement.EquallySpacedRectSide\",\"uuid\":\"86f54ccf-23de-43ab-be63-92a8881a04a3\"}]},\"type\":\"ConnectorPlacement.EquallySpacedConnector\",\"uuid\":\"5c8192db-99f5-4e0b-9632-6c54e7eb95e2\"}],\"packageUris\":[\"http://schema.mathworks.com/mf0/Connector/R2020b\"],\"version\":\"1.0\"}"
  discreteController7 : Subsystem
      settings: PortSchema="{\"entries\":[{\"content\":{\"sides\":[{\"content\":{\"connectorIds\":[\"In1\"]},\"type\":\"ConnectorPlacement.EquallySpacedRectSide\",\"uuid\":\"c21bf5a5-0def-4d0b-a33c-ffee9b3485af\"},{\"content\":{\"connectorIds\":[\"Out1\"],\"side\":\"RIGHT\"},\"type\":\"ConnectorPlacement.EquallySpacedRectSide\",\"uuid\":\"821ecc78-a01a-44e5-a9eb-88440e9f59ac\"},{\"content\":{\"connectorIds\":[],\"side\":\"TOP\"},\"type\":\"ConnectorPlacement.EquallySpacedRectSide\",\"uuid\":\"8999c1fd-a485-4668-b36c-e9eed9eb6d51\"},{\"content\":{\"connectorIds\":[\"In2\"],\"side\":\"BOTTOM\"},\"type\":\"ConnectorPlacement.EquallySpacedRectSide\",\"uuid\":\"a6e4704b-9925-4d06-9ffd-ba41902e8aa3\"},{\"content\":{\"connectorIds\":[],\"side\":\"HIDDEN\"},\"type\":\"ConnectorPlacement.EquallySpacedRectSide\",\"uuid\":\"86f54ccf-23de-43ab-be63-92a8881a04a3\"}]},\"type\":\"ConnectorPlacement.EquallySpacedConnector\",\"uuid\":\"5c8192db-99f5-4e0b-9632-6c54e7eb95e2\"}],\"packageUris\":[\"http://schema.mathworks.com/mf0/Connector/R2020b\"],\"version\":\"1.0\"}"
  discreteController8 : Subsystem
      settings: PortSchema="{\"entries\":[{\"content\":{\"sides\":[{\"content\":{\"connectorIds\":[\"In1\"]},\"type\":\"ConnectorPlacement.EquallySpacedRectSide\",\"uuid\":\"c21bf5a5-0def-4d0b-a33c-ffee9b3485af\"},{\"content\":{\"connectorIds\":[\"Out1\"],\"side\":\"RIGHT\"},\"type\":\"ConnectorPlacement.EquallySpacedRectSide\",\"uuid\":\"821ecc78-a01a-44e5-a9eb-88440e9f59ac\"},{\"content\":{\"connectorIds\":[],\"side\":\"TOP\"},\"type\":\"ConnectorPlacement.EquallySpacedRectSide\",\"uuid\":\"8999c1fd-a485-4668-b36c-e9eed9eb6d51\"},{\"content\":{\"connectorIds\":[\"In2\"],\"side\":\"BOTTOM\"},\"type\":\"ConnectorPlacement.EquallySpacedRectSide\",\"uuid\":\"a6e4704b-9925-4d06-9ffd-ba41902e8aa3\"},{\"content\":{\"connectorIds\":[],\"side\":\"HIDDEN\"},\"type\":\"ConnectorPlacement.EquallySpacedRectSide\",\"uuid\":\"86f54ccf-23de-43ab-be63-92a8881a04a3\"}]},\"type\":\"ConnectorPlacement.EquallySpacedConnector\",\"uuid\":\"5c8192db-99f5-4e0b-9632-6c54e7eb95e2\"}],\"packageUris\":[\"http://schema.mathworks.com/mf0/Connector/R2020b\"],\"version\":\"1.0\"}"
  Out1 : Outport
  wires:
  Sum/1 -> PID Controller/1
  PID Controller/1 -> Sum1/2
  Step/1 -> Scope/2, Gain/1, Sum/1  "ref"
  Transfer Fcn/1 -> Scope/1, Sum/2  "output"
  Gain/1 -> Transfer Fcn2/1
  Sum1/1 -> Saturation/1, Scope1/1  "u"
  Saturation/1 -> Scope1/2, Transfer Fcn/1  "sat_u"
  Transfer Fcn2/1 -> Sum1/1
  Transfer Fcn3/1 -> Sum2/1
  Gain1/1 -> Transfer Fcn3/1
  Sum3/1 -> Subsystem/1(e)
  Subsystem/1(u) -> Sum2/2
  Transfer Fcn1/1 -> Scope2/2, Sum3/2, Subsystem/2(fb)  "output_5"
  Saturation1/1 -> Transfer Fcn1/1, Scope3/2  "sat_u"
  Sum2/1 -> Scope3/1, Saturation1/1  "u"
  Saturation2/1 -> Transfer Fcn4/1, Scope4/2  "sat_u"
  Sum4/1 -> Scope4/1, Saturation2/1  "u"
  Subsystem1/1(u) -> Sum4/2
  Transfer Fcn4/1 -> Sum5/2, Subsystem1/2(fb), Scope2/3  "output_7"
  Sum5/1 -> Subsystem1/1(e)
  Sum7/1 -> Subsystem2/1(e)
  Transfer Fcn5/1 -> Subsystem2/2(fb), Sum7/2, Scope2/4  "output_3"
  Subsystem2/1(u) -> Sum6/2
  Sum6/1 -> Saturation3/1, Scope5/1  "u"
  Saturation3/1 -> Scope5/2, Transfer Fcn5/1  "sat_u"
  Saturation4/1 -> Transfer Fcn6/1, Scope6/2  "sat_u"
  Sum8/1 -> Scope6/1, Saturation4/1  "u"
  Subsystem3/1(u) -> Sum8/2
  Transfer Fcn6/1 -> Sum9/2, Subsystem3/2(fb), Scope2/5  "output_1"
  Step1/1 -> Scope2/1, Sum3/1, Gain1/1, Sum9/1, Sum7/1, Sum5/1  "ref"
  Sum9/1 -> Subsystem3/1(e)
  Saturation5/1 -> Transfer Fcn7/1, Scope7/2  "sat_u"
  Sum10/1 -> Scope7/1, Saturation5/1  "u"
  ? -> ?  "ref"
  Transfer Fcn7/1 -> 431throttle2wrpm/1(u)  "output_5"
  Subsystem5/1(u) -> Sum10/2
  Sum11/1 -> Subsystem5/1(e)
  431wrpm2throttle1/1(y) -> Sum10/1, Sum11/1  "ref_throttle"
  431wrpm2throttle/1(y) -> Subsystem5/2(fb), Sum11/2
  431throttle2wrpm/1(y) -> 431wrpm2throttle/1(u), Scope8/2
  Sum13/1 -> Subsystem6/1(e)
  430wrpm2throttle2/1(y) -> Subsystem6/2(fb), Sum13/2
  Transfer Fcn9/1 -> 430throttle2wrpm1/1(u)  "output_5"
  Saturation6/1 -> Transfer Fcn9/1, Scope9/2  "sat_u"
  Sum12/1 -> Scope9/1, Saturation6/1  "u"
  430throttle2wrpm1/1(y) -> 430wrpm2throttle2/1(u), Scope8/3
  Subsystem6/1(u) -> Sum12/2
  430wrpm2throttle3/1(y) -> Sum12/1, Sum13/1  "ref_throttle"
  429wrpm2throttle4/1(y) -> Sum14/1, Sum15/1  "ref_throttle"
  Subsystem7/1(u) -> Sum14/2
  Sum14/1 -> Scope10/1, Saturation7/1  "u"
  429wrpm2throttle1/1(y) -> Subsystem7/2(fb), Sum15/2
  429throttle2wrpm2/1(y) -> 429wrpm2throttle1/1(u), Scope8/4
  Saturation7/1 -> Transfer Fcn10/1, Scope10/2  "sat_u"
  Sum15/1 -> Subsystem7/1(e)
  Transfer Fcn10/1 -> 429throttle2wrpm2/1(u)  "output_5"
  Transfer Fcn11/1 -> 428throttle2wrpm1/1(u)  "output_5"
  Sum17/1 -> Subsystem8/1(e)
  Saturation8/1 -> Scope11/2, Transfer Fcn11/1  "sat_u"
  428throttle2wrpm1/1(y) -> 428wrpm2throttle2/1(u), Scope8/5
  428wrpm2throttle2/1(y) -> Sum17/2, Subsystem8/2(fb)
  Sum16/1 -> Saturation8/1, Scope11/1  "u"
  Subsystem8/1(u) -> Sum16/2
  428wrpm2throttle3/1(y) -> Sum17/1, Sum16/1  "ref_throttle"
  427wrpm2throttle4/1(y) -> Sum18/1, Sum19/1  "ref_throttle"
  Subsystem9/1(u) -> Sum18/2
  Sum18/1 -> Scope12/1, Saturation9/1  "u"
  427wrpm2throttle1/1(y) -> Subsystem9/2(fb), Sum19/2
  427throttle2wrpm2/1(y) -> 427wrpm2throttle1/1(u), Scope8/6
  Saturation9/1 -> Transfer Fcn12/1, Scope12/2  "sat_u"
  Sum19/1 -> Subsystem9/1(e)
  Transfer Fcn12/1 -> 427throttle2wrpm2/1(u)  "output_5"
  Transfer Fcn13/1 -> 426throttle2wrpm1/1(u)  "output_5"
  Sum21/1 -> Subsystem10/1(e)
  Saturation10/1 -> Scope13/2, Transfer Fcn13/1  "sat_u"
  426throttle2wrpm1/1(y) -> 426wrpm2throttle2/1(u), Scope8/7
  426wrpm2throttle2/1(y) -> Sum21/2, Subsystem10/2(fb)
  Sum20/1 -> Saturation10/1, Scope13/1  "u"
  Subsystem10/1(u) -> Sum20/2
  426wrpm2throttle3/1(y) -> Sum21/1, Sum20/1  "ref_throttle"
  Step2/1 -> 428wrpm2throttle3/1(u), 013wrpm2throttle3/1(u), 015wrpm2throttle4/1(u), 426wrpm2throttle3/1(u), 427wrpm2throttle4/1(u), 429wrpm2throttle4/1(u), 430wrpm2throttle3/1(u), Scope8/1, 431wrpm2throttle1/1(u)  "ref"
  015wrpm2throttle4/1(y) -> Sum23/1, Sum22/1  "ref_throttle"
  015throttle2wrpm2/1(y) -> 015wrpm2throttle1/1(u), Scope8/8
  Sum22/1 -> Saturation11/1, Scope14/1  "u"
  Saturation11/1 -> Scope14/2, Transfer Fcn14/1  "sat_u"
  Subsystem11/1(u) -> Sum22/2
  Transfer Fcn14/1 -> 015throttle2wrpm2/1(u)  "output_5"
  Sum23/1 -> Subsystem11/1(e)
  015wrpm2throttle1/1(y) -> Sum23/2, Subsystem11/2(fb)
  Saturation12/1 -> Scope15/2, Transfer Fcn15/1  "sat_u"
  Subsystem12/1(u) -> Sum24/2
  013wrpm2throttle2/1(y) -> Sum25/2, Subsystem12/2(fb)
  Sum25/1 -> Subsystem12/1(e)
  Sum24/1 -> Saturation12/1, Scope15/1  "u"
  Transfer Fcn15/1 -> 013throttle2wrpm1/1(u)  "output_5"
  013wrpm2throttle3/1(y) -> Sum25/1, Sum24/1  "ref_throttle"
  013throttle2wrpm1/1(y) -> 013wrpm2throttle2/1(u), Scope8/9
  013throttle2wrpm2/1(y) -> 427wrpm2throttle2/1(u), Scope23/10
  427wrpm2throttle3/1(y) -> Sum40/1, Sum41/1  "ref_throttle"
  Transfer Fcn21/1 -> 013throttle2wrpm2/1(u)  "output_5"
  Sum40/1 -> Scope21/1, Saturation15/1  "u"
  Sum41/1 -> Subsystem15/1(e)
  427wrpm2throttle2/1(y) -> Subsystem15/2(fb), Sum41/2
  Subsystem15/1(u) -> Sum40/2
  Saturation15/1 -> Transfer Fcn21/1, Scope21/2  "sat_u"
  427wrpm2throttle5/1(y) -> Subsystem13/2(fb), Sum39/2
  Sum39/1 -> Subsystem13/1(e)
  Transfer Fcn20/1 -> 015throttle2wrpm1/1(u)  "output_5"
  Subsystem13/1(u) -> Sum38/2
  Saturation14/1 -> Transfer Fcn20/1, Scope20/2  "sat_u"
  Sum38/1 -> Scope20/1, Saturation14/1  "u"
  015throttle2wrpm1/1(y) -> 427wrpm2throttle5/1(u), Scope23/9
  427wrpm2throttle6/1(y) -> Transfer Fcn29/1, Sum39/1  "ref_throttle"
  Step3/1 -> 427wrpm2throttle17/1(u), Transfer Fcn24/1, Scope23/2, 427wrpm2throttle15/1(u), 427wrpm2throttle13/1(u), 427wrpm2throttle11/1(u), 427wrpm2throttle9/1(u), 427wrpm2throttle7/1(u), 427wrpm2throttle6/1(u), 427wrpm2throttle3/1(u)  "ref"
  427wrpm2throttle7/1(y) -> Transfer Fcn28/1, Sum37/1  "ref_throttle"
  Subsystem22/1(u) -> Sum36/2
  Sum36/1 -> Scope19/1, Saturation13/1  "u"
  427wrpm2throttle8/1(y) -> Sum37/2, Subsystem22/2(fb)
  426throttle2wrpm2/1(y) -> 427wrpm2throttle8/1(u), Scope23/8
  Saturation13/1 -> Transfer Fcn19/1, Scope19/2  "sat_u"
  Sum37/1 -> Subsystem22/1(e)
  Transfer Fcn19/1 -> 426throttle2wrpm2/1(u)  "output_5"
  Transfer Fcn18/1 -> 427throttle2wrpm1/1(u)  "output_5"
  Sum35/1 -> Subsystem14/1(e)
  Saturation20/1 -> Scope18/2, Transfer Fcn18/1  "sat_u"
  427throttle2wrpm1/1(y) -> 427wrpm2throttle10/1(u), Scope23/7
  427wrpm2throttle10/1(y) -> Subsystem14/2(fb), Sum35/2
  Sum34/1 -> Saturation20/1, Scope18/1  "u"
  Subsystem14/1(u) -> Sum34/2
  427wrpm2throttle9/1(y) -> Sum35/1, Sum34/1  "ref_throttle"
  427wrpm2throttle11/1(y) -> Sum32/1, Sum33/1  "ref_throttle"
  Subsystem19/1(u) -> Sum32/2
  Sum32/1 -> Scope17/1, Saturation19/1  "u"
  427wrpm2throttle12/1(y) -> Subsystem19/2(fb), Sum33/2
  428throttle2wrpm2/1(y) -> 427wrpm2throttle12/1(u), Scope23/6
  Saturation19/1 -> Transfer Fcn17/1, Scope17/2  "sat_u"
  Sum33/1 -> Subsystem19/1(e)
  Transfer Fcn17/1 -> 428throttle2wrpm2/1(u)  "output_5"
  Transfer Fcn16/1 -> 429throttle2wrpm1/1(u)  "output_5"
  Sum31/1 -> Subsystem18/1(e)
  Saturation18/1 -> Scope16/2, Transfer Fcn16/1  "sat_u"
  429throttle2wrpm1/1(y) -> 427wrpm2throttle14/1(u), Scope23/5
  427wrpm2throttle14/1(y) -> Subsystem18/2(fb), Sum31/2
  Sum30/1 -> Saturation18/1, Scope16/1  "u"
  Subsystem18/1(u) -> Sum30/2
  427wrpm2throttle13/1(y) -> Sum31/1, Transfer Fcn27/1  "ref_throttle"
  427wrpm2throttle15/1(y) -> Sum29/1, Transfer Fcn26/1  "ref_throttle"
  Subsystem17/1(u) -> Sum28/2
  430throttle2wrpm2/1(y) -> 427wrpm2throttle16/1(u), Scope23/4
  Sum28/1 -> Saturation17/1, Scope24/1  "u"
  Saturation17/1 -> Scope24/2, Transfer Fcn23/1  "sat_u"
  Transfer Fcn23/1 -> 430throttle2wrpm2/1(u)  "output_5"
  427wrpm2throttle16/1(y) -> Subsystem17/2(fb), Sum29/2
  Sum29/1 -> Subsystem17/1(e)
  431throttle2wrpm1/1(y) -> 427wrpm2throttle18/1(u), Scope23/3
  427wrpm2throttle18/1(y) -> Sum27/2, Subsystem16/2(fb)
  427wrpm2throttle17/1(y) -> Sum27/1, Transfer Fcn25/1  "ref_throttle"
  Sum27/1 -> Subsystem16/1(e)
  Subsystem16/1(u) -> Sum26/2
  Transfer Fcn22/1 -> 431throttle2wrpm1/1(u)  "output_5"
  Sum26/1 -> Saturation16/1, Scope22/1  "u"
  Saturation16/1 -> Scope22/2, Transfer Fcn22/1  "sat_u"
  Transfer Fcn24/1 -> Scope23/1  "compare"
  Transfer Fcn25/1 -> Sum26/1  "compare"
  Transfer Fcn26/1 -> Sum28/1  "compare"
  Transfer Fcn27/1 -> Sum30/1  "compare"
  Transfer Fcn28/1 -> Sum36/1  "compare"
  Transfer Fcn29/1 -> Sum38/1  "compare"
  Discrete Transfer Fcn7/1 -> Sum54/1  "compare"
  Discrete Transfer Fcn6/1 -> Sum52/1  "compare"
  Discrete Transfer Fcn3/1 -> Sum46/1  "compare"
  Discrete Transfer Fcn2/1 -> Sum44/1  "compare"
  Gain2/1 -> Discrete Transfer Fcn1/1  "compare"
  Transfer Fcn38/1 -> Scope32/1  "compare"
  Saturation24/1 -> Discrete Transfer Fcn9/1, Transport Delay2/1, Scope31/2  "sat_u"
  Sum42/1 -> Scope31/1, Saturation24/1  "u"
  Transfer Fcn36/1 -> 428throttle2wrpm4/1(u)  "output_5"
  discreteController8/1(u) -> Sum42/2
  427wrpm2throttle26/1(y) -> Sum43/1, Gain2/1  "ref_throttle"
  Sum45/1 -> discreteController1/1(e)
  427wrpm2throttle25/1(y) -> discreteController1/2(fb), Sum45/2
  Transfer Fcn37/1 -> 430throttle2wrpm3/1(u)  "output_5"
  Saturation25/1 -> Transfer Fcn37/1, Scope33/2  "sat_u"
  Sum44/1 -> Scope33/1, Saturation25/1  "u"
  430throttle2wrpm3/1(y) -> Scope32/4, 427wrpm2throttle25/1(u)
  discreteController1/1(u) -> Sum44/2
  427wrpm2throttle24/1(y) -> Discrete Transfer Fcn2/1, Sum45/1  "ref_throttle"
  427wrpm2throttle22/1(y) -> Discrete Transfer Fcn3/1, Sum47/1  "ref_throttle"
  discreteController2/1(u) -> Sum46/2
  Sum46/1 -> Scope25/1, Saturation26/1  "u"
  427wrpm2throttle23/1(y) -> discreteController2/2(fb), Sum47/2
  429throttle2wrpm3/1(y) -> Scope32/5, 427wrpm2throttle23/1(u)
  Saturation26/1 -> Transfer Fcn30/1, Scope25/2  "sat_u"
  Sum47/1 -> discreteController2/1(e)
  Transfer Fcn30/1 -> 429throttle2wrpm3/1(u)  "output_5"
  Transfer Fcn31/1 -> 428throttle2wrpm3/1(u)  "output_5"
  Sum49/1 -> discreteController3/1(e)
  Saturation27/1 -> Scope26/2, Transfer Fcn31/1  "sat_u"
  428throttle2wrpm3/1(y) -> Scope32/6, 427wrpm2throttle21/1(u)
  427wrpm2throttle21/1(y) -> Sum49/2, discreteController3/2(fb)
  Sum48/1 -> Saturation27/1, Scope26/1  "u"
  discreteController3/1(u) -> Sum48/2
  427wrpm2throttle20/1(y) -> Sum49/1, Discrete Transfer Fcn4/1  "ref_throttle"
  427wrpm2throttle34/1(y) -> Discrete Transfer Fcn5/1, Sum51/1  "ref_throttle"
  discreteController4/1(u) -> Sum50/2
  Sum50/1 -> Scope27/1, Saturation28/1  "u"
  427wrpm2throttle19/1(y) -> discreteController4/2(fb), Sum51/2
  427throttle2wrpm3/1(y) -> Scope32/7, 427wrpm2throttle19/1(u)
  Saturation28/1 -> Transfer Fcn32/1, Scope27/2  "sat_u"
  Sum51/1 -> discreteController4/1(e)
  Transfer Fcn32/1 -> 427throttle2wrpm3/1(u)  "output_5"
  Transfer Fcn33/1 -> 426throttle2wrpm3/1(u)  "output_5"
  Sum53/1 -> discreteController5/1(e)
  Saturation21/1 -> Scope28/2, Transfer Fcn33/1  "sat_u"
  426throttle2wrpm3/1(y) -> Scope32/8, 427wrpm2throttle33/1(u)
  427wrpm2throttle33/1(y) -> discreteController5/2(fb), Sum53/2
  Sum52/1 -> Saturation21/1, Scope28/1  "u"
  discreteController5/1(u) -> Sum52/2
  427wrpm2throttle32/1(y) -> Discrete Transfer Fcn6/1, Sum53/1  "ref_throttle"
  Step4/1 -> Scope32/2, Transport Delay3/1, 427wrpm2throttle26/1(u), 427wrpm2throttle29/1(u), 427wrpm2throttle31/1(u), 427wrpm2throttle32/1(u), 427wrpm2throttle34/1(u), 427wrpm2throttle20/1(u), 427wrpm2throttle22/1(u), 427wrpm2throttle24/1(u)  "ref"
  427wrpm2throttle31/1(y) -> Discrete Transfer Fcn7/1, Sum55/1  "ref_throttle"
  015throttle2wrpm3/1(y) -> Scope32/9, 427wrpm2throttle30/1(u)
  Sum54/1 -> Saturation22/1, Scope29/1  "u"
  Saturation22/1 -> Scope29/2, Transfer Fcn34/1  "sat_u"
  discreteController6/1(u) -> Sum54/2
  Transfer Fcn34/1 -> 015throttle2wrpm3/1(u)  "output_5"
  Sum55/1 -> discreteController6/1(e)
  427wrpm2throttle30/1(y) -> discreteController6/2(fb), Sum55/2
  Saturation23/1 -> Scope30/2, Transfer Fcn35/1  "sat_u"
  discreteController7/1(u) -> Sum56/2
  427wrpm2throttle28/1(y) -> discreteController7/2(fb), Sum57/2
  Sum57/1 -> discreteController7/1(e)
  Sum56/1 -> Saturation23/1, Scope30/1  "u"
  Transfer Fcn35/1 -> 013throttle2wrpm3/1(u)  "output_5"
  427wrpm2throttle29/1(y) -> Sum57/1, Discrete Transfer Fcn8/1  "ref_throttle"
  013throttle2wrpm3/1(y) -> Scope32/10, 427wrpm2throttle28/1(u)
  Discrete Transfer Fcn4/1 -> Sum48/1  "compare"
  Discrete Transfer Fcn5/1 -> Sum50/1  "compare"
  Discrete Transfer Fcn8/1 -> Sum56/1  "compare"
  In1/1 -> Sum59/1, Discrete Transfer Fcn10/1  "ref_throttle"
  Sum59/1 -> discreteController10/1(e)
  discreteController10/1(u) -> Sum58/2
  Discrete Transfer Fcn11/1 -> Out1/1, Sum59/2, discreteController10/2(fb)  "output_5"
  Sum58/1 -> Saturation29/1, Scope35/1  "u"
  Saturation29/1 -> Scope35/2, Discrete Transfer Fcn11/1  "sat_u"
  Discrete Transfer Fcn10/1 -> Sum58/1  "compare"
  428throttle2wrpm4/1(y) -> Scope32/3, 427wrpm2throttle27/1(u)
  Transport Delay2/1 -> Transfer Fcn36/1
  Discrete Transfer Fcn9/1 -> Sum60/1, Transport Delay1/1
  Transport Delay1/1 -> Sum60/2
  Transport Delay3/1 -> Transfer Fcn38/1
  Discrete Transfer Fcn1/1 -> Sum42/1  "compare"
  Sum43/1 -> Sum61/1
  Sum61/1 -> discreteController8/1(e)
  427wrpm2throttle27/1(y) -> Sum43/2
  Sum60/1 -> Sum61/2  "u"
